simulink model "REALTIME_PART2_errorspace"  (R2020b)
settings: Solver=ode3  StartTime=0.0  StopTime=5  FixedStep=0.001  RelTol=1e-3
undefined symbols (not defined in the file): Ar, degs2rpm, denH1, Kz, National_Instruments, numH1, PCI, rpm2rads, sens, step_size, Tr, w0
libraries: sldrtlib x2
settings Model: ExtModeTrigDuration=11000  Creator=utente  LastModifiedBy=ambrosingi
settings DataIOCC: ReturnWorkspaceOutputs=off
settings RTWCC: Description=Simulink Desktop Real-Time  SystemTargetFile=sldrt.tlc  TemplateMakefile=sldrt.tmf  RTWCompilerOptimization=on
settings CodeAppCC: MaxIdLength=95
settings SimulinkDesktopRealTimeCC: TargetPreCompLibLocation=C:\Program Files\MATLAB\R2020b\toolbox\sldrt\lib\win64

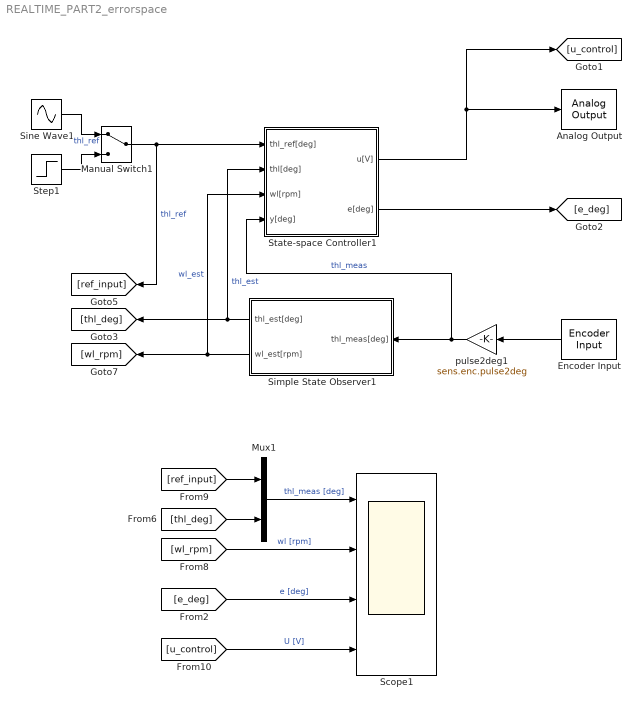
== system REALTIME_PART2_errorspace ==
  Analog Output : sldrtlib/Analog Output  SampleTime=0.001  MaxMissedTicks=10  ShowMissedTicks=off  YieldWhenWaiting=off  DrvName=National_Instruments/PCI-6221  DrvAddress=4294967295  DrvOptions=[0 0 0 2 0]  Channels=1  RangeMode=1  VoltRange=1  InitialValue=0  FinalValue=0
      settings: AttributesFormatString=National Instruments\nPCI-6221 [auto]
  Encoder Input : sldrtlib/Encoder Input  SampleTime=0.001  MaxMissedTicks=10  ShowMissedTicks=off  YieldWhenWaiting=off  DrvName=National_Instruments/PCI-6221  DrvAddress=4294967295  DrvOptions=[0 0 0 2 0]  Channels=1  QuadMode=3  IndexPulse=1  InputFilter=Inf  DataType=1
      settings: AttributesFormatString=National Instruments\nPCI-6221 [auto]
  Manual Switch1 : ManualSwitch
  Mux1 : Mux  Inputs=2
  Scope1 : Scope  NumInputPorts=4
  Simple State Observer1 : Subsystem
  Sine Wave1 : Sin  Amplitude=Ar  Frequency=2*pi/Tr  SampleTime=0
  State-space Controller1 : Subsystem
  Step1 : Step  After=step_size  SampleTime=0
  pulse2deg1 : Gain  Gain=sens.enc.pulse2deg
  wires:
  Mux1/1 -> Scope1/1  "thl_meas [deg]"
  [wl_rpm] -> Scope1/2  "wl [rpm]"
  [ref_input] -> Mux1/1
  Simple State Observer1/1(thl_est[deg]) -> State-space Controller1/2(thl[deg]), [thl_deg]  "thl_est"
  Manual Switch1/1 -> State-space Controller1/1(thl_ref[deg]), [ref_input]  "thl_ref"
  Simple State Observer1/2(wl_est[rpm]) -> State-space Controller1/3(wl[rpm]), [wl_rpm]  "wl_est"
  [u_control] -> Scope1/4  "U [V]"
  Encoder Input/1 -> pulse2deg1/1
  [thl_deg] -> Mux1/2
  State-space Controller1/1(u[V]) -> [u_control], Analog Output/1
  pulse2deg1/1 -> State-space Controller1/4(y[deg]), Simple State Observer1/1(thl_meas[deg])  "thl_meas"
  Sine Wave1/1 -> Manual Switch1/1  "thl_ref"
  Step1/1 -> Manual Switch1/2
  State-space Controller1/2(e[deg]) -> [e_deg]
  [e_deg] -> Scope1/3  "e [deg]"

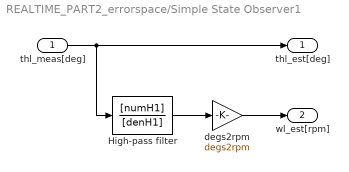
== system REALTIME_PART2_errorspace/Simple State Observer1 ==
  thl_meas[deg] : Inport
  High-pass filter : TransferFcn  Numerator=[numH1]  Denominator=[denH1]
  degs2rpm : Gain  Gain=degs2rpm
  thl_est[deg] : Outport
  wl_est[rpm] : Outport  Port=2
  wires:
  thl_meas[deg]/1 -> thl_est[deg]/1, High-pass filter/1
  High-pass filter/1 -> degs2rpm/1
  degs2rpm/1 -> wl_est[rpm]/1

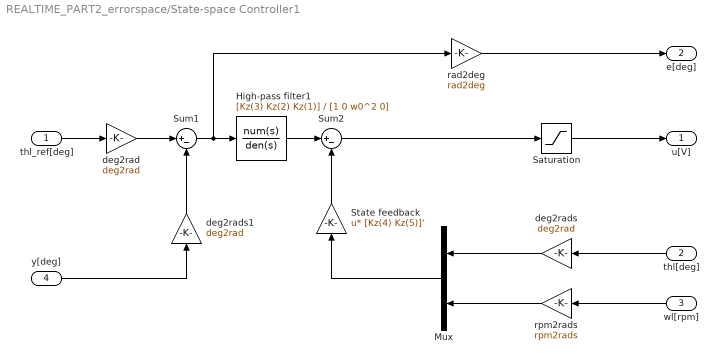
== system REALTIME_PART2_errorspace/State-space Controller1 ==
  thl_ref[deg] : Inport
  thl[deg] : Inport  Port=2
  wl[rpm] : Inport  Port=3
  y[deg] : Inport  Port=4
  High-pass filter1 : TransferFcn  Numerator=[Kz(3) Kz(2) Kz(1)]  Denominator=[1 0 w0^2 0]
  Mux : Mux  Inputs=2
  Saturation : Saturate  UpperLimit=10  LowerLimit=-10
  State feedback : Gain  Gain=[Kz(4) Kz(5)]'  Multiplication=Matrix(u*K)
  Sum1 : Sum  Inputs=|+-
  Sum2 : Sum  Inputs=|+-
  deg2rad : Gain  Gain=deg2rad
  deg2rads : Gain  Gain=deg2rad
  deg2rads1 : Gain  Gain=deg2rad
  rad2deg : Gain  Gain=rad2deg
  rpm2rads : Gain  Gain=rpm2rads
  u[V] : Outport
  e[deg] : Outport  Port=2
  wires:
  State feedback/1 -> Sum2/2
  Mux/1 -> State feedback/1
  High-pass filter1/1 -> Sum2/1
  Sum1/1 -> rad2deg/1, High-pass filter1/1
  deg2rads1/1 -> Sum1/2
  y[deg]/1 -> deg2rads1/1
  wl[rpm]/1 -> rpm2rads/1
  thl[deg]/1 -> deg2rads/1
  rpm2rads/1 -> Mux/2
  deg2rads/1 -> Mux/1
  deg2rad/1 -> Sum1/1
  thl_ref[deg]/1 -> deg2rad/1
  rad2deg/1 -> e[deg]/1
  Sum2/1 -> Saturation/1
  Saturation/1 -> u[V]/1
